simulink model "sschdlexFlybackConverterExample"  (R2023b)
settings: Solver=FixedStepDiscrete  StartTime=0.0  StopTime=200e-6  RelTol=1e-3
InitFcn:
  | ts = 2e-008;
libraries: fl_lib x13, nesl_utility x7, ee_lib x2, simulink x1, hdlsllib x1
CloseFcn:
  | clear ts;
settings Model: DataTypeOverride=Off  Creator=The MathWorks, Inc.  LastModifiedBy=The MathWorks, Inc.
settings SolverCC: AlgebraicLoopSolver=TrustRegion
settings OptimizationCC: BlockReduction=off  ConditionallyExecuteInputs=off  DefaultParameterBehavior=Inlined
settings DebuggingCC: AlgebraicLoopMsg=error  SingleTaskRateTransMsg=error  ParameterPrecisionLossMsg=none  UnconnectedInputMsg=warning  UnconnectedOutputMsg=warning  UnconnectedLineMsg=warning
settings HardwareCC: ProdBitPerPointer=32  ProdBitPerSizeT=32  ProdBitPerPtrDiffT=32  ProdLargestAtomicFloat=None  ProdIntDivRoundTo=Undefined  ProdEndianess=Unspecified  ProdWordSize=32  ProdHWDeviceType=ASIC/FPGA->ASIC/FPGA  TargetBitPerPointer=64  TargetBitPerSizeT=64  TargetBitPerPtrDiffT=64  TargetLongLongMode=on  TargetIntDivRoundTo=Zero  TargetEndianess=LittleEndian  TargetWordSize=64  TargetHWDeviceType=Custom Processor->MATLAB Host Computer  ProdEqTarget=off
settings ModelReferenceCC: EnableRefExpFcnMdlSchedulingChecks=on
settings RTWCC: DLArmComputeVersion=19.05

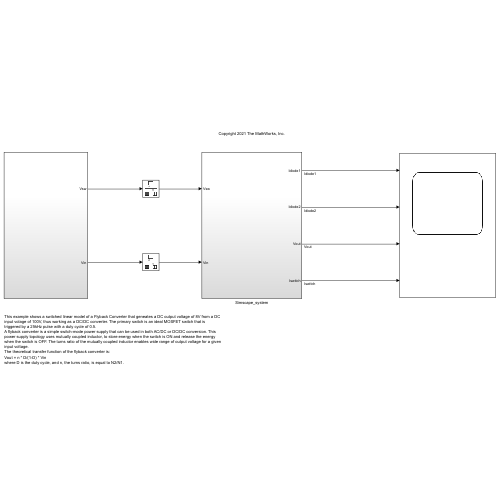
[thumbnail: Simulink's stored preview of the top-level diagram]
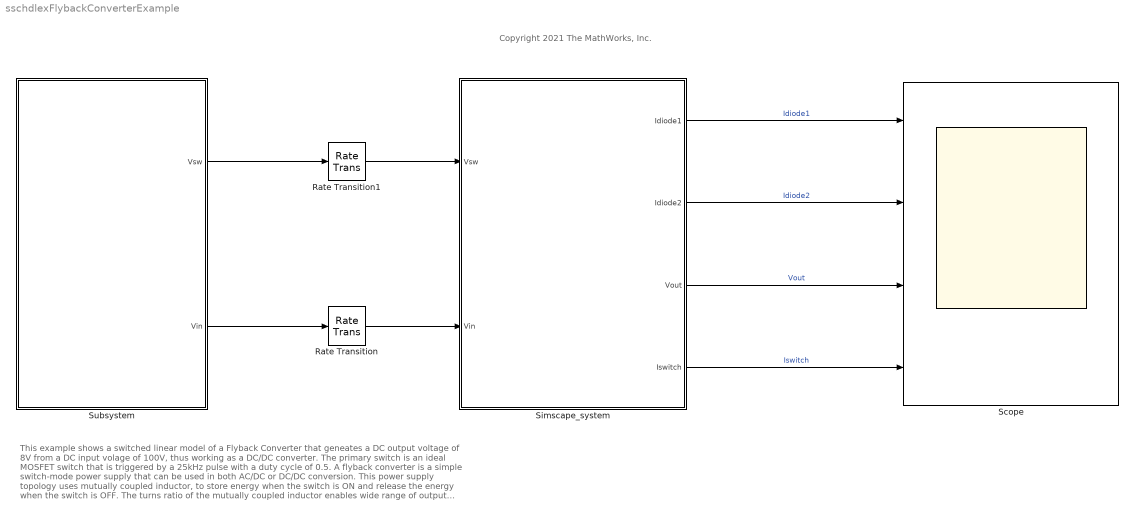
== system sschdlexFlybackConverterExample ==
  note: This example shows a switched linear model of a Flyback Converter that geneates a DC output voltage of 8V from a DC input volage of 100V, thus working as a DC/DC converter. The primary switch is an ideal MOSFET switch that is triggered by a 25kHz pulse with a duty cycle of 0.5.
      | A flyback converter is a simple switch-mode power supply that can be used in both AC/DC or DC/DC conversion. This power supply topology uses mutually coupled inductor, to store energy when the switch is ON and release the energy when the switch is OFF. The turns ratio of the mutually coupled inductor enables wide range of output voltage for a given input voltage.
      | The theoretical transfer function of the flyback converter is:
      | Vout = n * D/(1-D) * Vin
      | where D is the duty cycle, and n, the turns ratio, is equal to N2/N1.
  note: Copyright 2021 The MathWorks, Inc.
  Rate Transition : RateTransition
  Rate Transition1 : RateTransition
  Scope : Scope  NumInputPorts=4
  Simscape_system : Subsystem
  Subsystem : Subsystem
  wires:
  Subsystem/1(Vsw) -> Rate Transition1/1
  Subsystem/2(Vin) -> Rate Transition/1
  Rate Transition1/1 -> Simscape_system/1(Vsw)
  Rate Transition/1 -> Simscape_system/2(Vin)
  Simscape_system/1(Idiode1) -> Scope/1  "Idiode1"
  Simscape_system/2(Idiode2) -> Scope/2  "Idiode2"
  Simscape_system/3(Vout) -> Scope/3  "Vout"
  Simscape_system/4(Iswitch) -> Scope/4  "Iswitch"

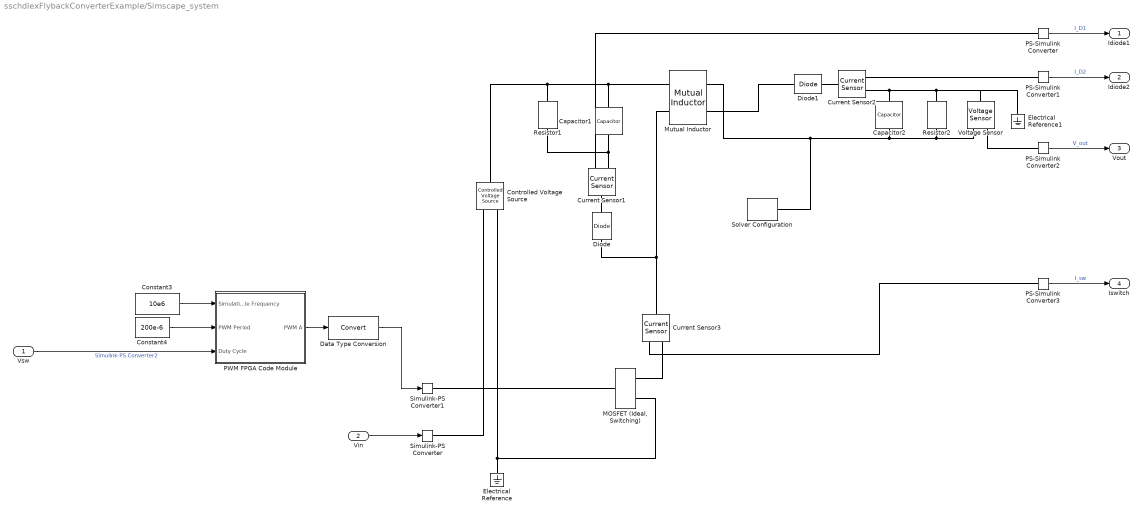
== system sschdlexFlybackConverterExample/Simscape_system ==
  Vsw : Inport
  Vin : Inport  Port=2
  Capacitor1 : fl_lib/Electrical/Electrical Elements/Capacitor  c=0.1e-12 F  r=0 Ohm  g=0 1/Ohm  i_specify=off  i_priority=None  i=0 A  i_nominal_specify=off  i_nominal_unit=A  i_nominal_value=1  v_specify=off  v_priority=None  v=0 V  v_nominal_specify=off  v_nominal_unit=V  v_nominal_value=1  vc_specify=off  vc_priority=High  vc=0 V  vc_nominal_specify=off  vc_nominal_unit=V  vc_nominal_value=1
  Capacitor2 : fl_lib/Electrical/Electrical Elements/Capacitor  c=50e-6 F  r=0 Ohm  g=0 1/Ohm  i_specify=off  i_priority=None  i=0 A  i_nominal_specify=off  i_nominal_unit=A  i_nominal_value=1  v_specify=off  v_priority=None  v=0 V  v_nominal_specify=off  v_nominal_unit=V  v_nominal_value=1  vc_specify=on  vc_priority=High  vc=8 V  vc_nominal_specify=off  vc_nominal_unit=V  vc_nominal_value=1
  Constant3 : Constant  Value=10e6  OutDataTypeStr=single  SampleTime=-1
  Constant4 : Constant  Value=200e-6  OutDataTypeStr=single  SampleTime=-1
  Controlled Voltage Source : fl_lib/Electrical/Electrical Sources/Controlled Voltage Source
  Current Sensor1 : fl_lib/Electrical/Electrical Sensors/Current Sensor
  Current Sensor2 : fl_lib/Electrical/Electrical Sensors/Current Sensor
  Current Sensor3 : fl_lib/Electrical/Electrical Sensors/Current Sensor
  Data Type Conversion : DataTypeConversion  SaturateOnIntegerOverflow=off  RndMeth=Floor
  Diode : fl_lib/Electrical/Electrical Elements/Diode  Vf=0.001 V  Ron=0.001 Ohm  Goff=1e-6 1/Ohm  i_specify=off  i_priority=None  i=0 A  i_nominal_specify=off  i_nominal_unit=A  i_nominal_value=1  v_specify=off  v_priority=None  v=0 V  v_nominal_specify=off  v_nominal_unit=V  v_nominal_value=1
  Diode1 : fl_lib/Electrical/Electrical Elements/Diode  Vf=0.25 V  Ron=0.3 Ohm  Goff=1e-8 1/Ohm  i_specify=off  i_priority=None  i=0 A  i_nominal_specify=off  i_nominal_unit=A  i_nominal_value=1  v_specify=off  v_priority=None  v=0 V  v_nominal_specify=off  v_nominal_unit=V  v_nominal_value=1
  Electrical Reference : fl_lib/Electrical/Electrical Elements/Electrical Reference
  Electrical Reference1 : fl_lib/Electrical/Electrical Elements/Electrical Reference
  "MOSFET (Ideal, Switching)" : ee_lib/Semiconductors & Converters/MOSFET (Ideal, Switching)  Rds=1e-9 Ohm  Goff=1e-9 1/Ohm  Vth=0.001 V  diode_param=1  diode_Vf=0.8 V  diode_Ron=0.001 Ohm  diode_Goff=1e-5 1/Ohm  diode_C=50e-9 F  diode_iRM=-235 A  diode_iF=300 A  diode_idot=-50 A/us  diode_trr_param=1  diode_trr_factor=3  diode_trr=15 us  diode_Qrr=1500 s*uA  thermal_loss_option=ee.enum.converters.thermalLossOption.constantvalues  Von_data=[0, 1.1, 1.3, 1.45, 1.75, 2.25, 2.7; 0, 1, 1.15, 1.35, 1.7, 2.35, 3] V  Eon_data=[0, .29, 1.43, 2.86, 5.71, 13.14, 22.86; 0, .57, 2.63, 5.14, 10.29, 20.57, 30.29] * 1e-3 J  Eoff_data=[0, .21, 1.07, 2.14, 4.29, 9.86, 17.14; 0, .43, 1.97, 3.86, 7.71, 15.43, 22.71] * 1e-3 J  Tj=[298.15, 398.15] K  Iout_data=[0, 10, 50, 100, 200, 400, 600] A  Eon_scalar=22.86e-3 J  Eoff_scalar=17.14e-3 J  Voff=300 V  Iout_scalar=600 A  diodeModelType=ee.enum.converters.diodeModelType.pwl  diode_IfMat=[.07, .12, .19, 1.75, 4.24, 7.32, 11.2; .16, .3, .72, 2.14, 4.02, 6.35, 9.12] A  diode_TjVec=[25, 125] degC  diode_VfVec=[.5, .7, .9, 1.3, 1.7, 2.1, 2.5] V  thermal_network_parameterization=ee.enum.thermalNetworkTopology.external  Rth=[.03, .2] K/W  Rth_Foster=[.03, .2] K/W  thermal_mass_parameterization=ee.enum.thermalNetwork.timeconstant  thermal_mass=[3, 25] J/K  thermal_mass_Foster=[33, 50] J/K  thermal_time_constant=[.1, 5] s  thermal_time_constant_Foster=[1, 10] s  thermal_mass_initial_temperatures=[25, 25] degC  junction_thermal_mass=0.1 J/K  Tau=1e-4 s  vT_specify=off  vT_priority=None  vT=0 V  vT_nominal_specify=off  vT_nominal_unit=V  vT_nominal_value=1  Qj_specify=off  Qj_priority=None  Qj=0 W  Qj_nominal_specify=off  Qj_nominal_unit=W  Qj_nominal_value=1  junction_temperature_specify=off  junction_temperature_priority=None  junction_temperature=25 degC  junction_temperature_nominal_specify=off  junction_temperature_nominal_unit=degC  junction_temperature_nominal_value=1
  Mutual Inductor : ee_lib/Passive/Transformers/Mutual Inductor  L1=10 uH  L2=10 uH  k=0.08  L_tol=5  enable_L1_tol=0  L1_tol_distribution=1  L1_nSigma=4  enable_L2_tol=0  L2_tol_distribution=1  L2_nSigma=4  r=[.1e-3, .1e-3] Ohm  g=[1e-09, 1e-09] 1/Ohm  enable_operating_limits=0  operating_limit_action=2  max_working_current=1 A  power_rating=1 W  enable_faults=ee.enum.faults.faultEnable.no  fault_action=ee.enum.faults.faultAction.none  fault_winding=1  lambdaPercent=50  turnsShort=ee.enum.faults.faultTurnsShort.no  openCct=ee.enum.faults.faultTurnsOpenCkt.no  groundShort=ee.enum.faults.faultTurnsGroundShort.no  groundShortG=0 1/Ohm  tau_fault=1e-3 s  enable_temporal_fault=ee.enum.faults.faultTriggerTemporal.no  t_fault=1 s  enable_behavioral_fault=ee.enum.faults.faultTriggerBehavioral.no  max_permissible_voltage=100 V  n_fail_on_voltage=1  max_permissible_current=1 A  t_fail_on_current=1 s  iL1_specify=off  iL1_priority=High  iL1=0 A  iL1_nominal_specify=off  iL1_nominal_unit=A  iL1_nominal_value=1  iL2_specify=off  iL2_priority=High  iL2=0 A  iL2_nominal_specify=off  iL2_nominal_unit=A  iL2_nominal_value=1
      settings: InternalSimscapePortConfiguration="{\"Bottom\":[],\"Left\":[{\"id\":\"p1\",\"label\":\"1+\",\"type\":\"foundation.electrical.electrical\"},{\"id\":\"n1\",\"label\":\"1-\",\"type\":\"foundation.electrical.electrical\"}],\"Right\":[{\"id\":\"p2\",\"label\":\"2+\",\"type\":\"foundation.electrical.electrical\"},{\"id\":\"n2\",\"label\":\"2-\",\"type\":\"foundation.electrical.electrical\"}],\"Top\":[]}"
  PS-Simulink Converter{,1..3} (4 alike) : nesl_utility/PS-Simulink Converter  PhysicalDomain=network_engine_domain  SubClassName=ps_output  LeftPortType=input  RightPortType=output  PseudoPeriodic=off  Frequencies=[]  Unit=inherit  AffineConversion=off
  PWM FPGA Code Module : Subsystem  SystemSampleTime=1/75e6
  Resistor1 : fl_lib/Electrical/Electrical Elements/Resistor  R=50e3 Ohm  i_specify=off  i_priority=None  i=0 A  i_nominal_specify=off  i_nominal_unit=A  i_nominal_value=1  v_specify=off  v_priority=None  v=0 V  v_nominal_specify=off  v_nominal_unit=V  v_nominal_value=1
  Resistor2 : fl_lib/Electrical/Electrical Elements/Resistor  R=2.5 Ohm  i_specify=off  i_priority=None  i=0 A  i_nominal_specify=off  i_nominal_unit=A  i_nominal_value=1  v_specify=off  v_priority=None  v=0 V  v_nominal_specify=off  v_nominal_unit=V  v_nominal_value=1
  Simulink-PS Converter : nesl_utility/Simulink-PS Converter  PhysicalDomain=network_engine_domain  SubClassName=ps_input  LeftPortType=input  RightPortType=output  PseudoPeriodic=off  Frequencies=[]  NoiseDistribution=none  NoiseParameters=[]  Unit=1  AffineConversion=off  FilteringAndDerivatives=provide  SimscapeFilterOrder=1  InputFilterTimeConstant=0.001  UdotUserProvided=0
  Simulink-PS Converter1 : nesl_utility/Simulink-PS Converter  PhysicalDomain=network_engine_domain  SubClassName=ps_input  LeftPortType=input  RightPortType=output  PseudoPeriodic=off  Frequencies=[]  NoiseDistribution=none  NoiseParameters=[]  Unit=1  AffineConversion=off  FilteringAndDerivatives=provide  SimscapeFilterOrder=1  InputFilterTimeConstant=0.001  UdotUserProvided=0
  Solver Configuration : nesl_utility/Solver Configuration  PhysicalDomain=network_engine_domain  SubClassName=solver  LeftPortType=input  RightPortType=generic  Tones=[]  Harmonics=[]  SimulateNoise=off  Profile=off  UseLocalSampling=off  EnableSwitchedLinearOptims=on  FrequencyDomain=off  UseCCode=off  RelTol=0.001  AbsTol=1e-06  MinStep=1e-09  ToWorkspace=off  RevertToSquareIcSolve=off  NumHomotopyIterations=100  PhasorMode=off  PhasorModeNumHarmonics=1  DoDC=off  ResidualTolerance=1e-09  UseLocalSolver=on  LocalSolverChoice=NE_BACKWARD_EULER_ADVANCER  LocalSolverSampleTime=ts  DoFixedCost=on  MaxNonlinIter=3  MaxModeIter=2  ComputeImpulses=off  ImpulseIterations=1  LinearAlgebra=auto  EquationFormulation=NE_TIME_EF  DelaysMemoryBudget=1024  AutomaticFiltering=on  FilteringTimeConstant=0.001  PartitionStorageMethod=AS_NEEDED  PartitionMemoryBudget=1024  PartitionMethod=ROBUST
  Voltage Sensor : fl_lib/Electrical/Electrical Sensors/Voltage Sensor
  Idiode1 : Outport
  Idiode2 : Outport  Port=2
  Vout : Outport  Port=3
  Iswitch : Outport  Port=4
  wires:
  Data Type Conversion/1 -> Simulink-PS Converter1/1
  Vin/1 -> Simulink-PS Converter/1
  PS-Simulink Converter2/1 -> Vout/1  "V_out"
  PS-Simulink Converter1/1 -> Idiode2/1  "I_D2"
  PS-Simulink Converter/1 -> Idiode1/1  "I_D1"
  PS-Simulink Converter3/1 -> Iswitch/1  "I_sw"
  Vsw/1 -> PWM FPGA Code Module/3(Duty Cycle)  "Simulink-PS Converter2"
  Constant4/1 -> PWM FPGA Code Module/2(PWM Period)
  PWM FPGA Code Module/1(PWM A) -> Data Type Conversion/1
  Constant3/1 -> PWM FPGA Code Module/1(Simulation Sample Frequency)
  connections:
  Diode/RConn1 -- Current Sensor1/LConn1
  Electrical Reference/LConn1 -- "MOSFET (Ideal, Switching)"/RConn2 -- Controlled Voltage Source/RConn2
  "MOSFET (Ideal, Switching)"/LConn1 -- Simulink-PS Converter1/RConn1
  Capacitor1/RConn1 -- Resistor1/RConn1 -- Current Sensor1/RConn2
  Current Sensor3/LConn1 -- Diode/LConn1 -- Mutual Inductor/LConn2
  Current Sensor1/RConn1 -- PS-Simulink Converter/LConn1
  Diode1/RConn1 -- Current Sensor2/LConn1
  PS-Simulink Converter2/LConn1 -- Voltage Sensor/RConn1
  Current Sensor2/RConn2 -- Capacitor2/LConn1 -- Resistor2/LConn1 -- Electrical Reference1/LConn1 -- Voltage Sensor/LConn1
  Simulink-PS Converter/RConn1 -- Controlled Voltage Source/RConn1
  Controlled Voltage Source/LConn1 -- Resistor1/LConn1 -- Mutual Inductor/LConn1 -- Capacitor1/LConn1
  Solver Configuration/RConn1 -- Mutual Inductor/RConn1 -- Capacitor2/RConn1 -- Resistor2/RConn1 -- Voltage Sensor/RConn2
  PS-Simulink Converter1/LConn1 -- Current Sensor2/RConn1
  PS-Simulink Converter3/LConn1 -- Current Sensor3/RConn1
  Current Sensor3/RConn2 -- "MOSFET (Ideal, Switching)"/RConn1
  Diode1/LConn1 -- Mutual Inductor/RConn2

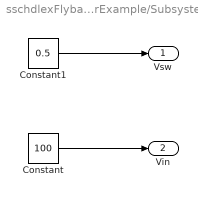
== system sschdlexFlybackConverterExample/Subsystem ==
  Constant : Constant  Value=100  SampleTime=0
  Constant1 : Constant  Value=0.5  SampleTime=ts
  Vsw : Outport
  Vin : Outport  Port=2
  wires:
  Constant1/1 -> Vsw/1
  Constant/1 -> Vin/1

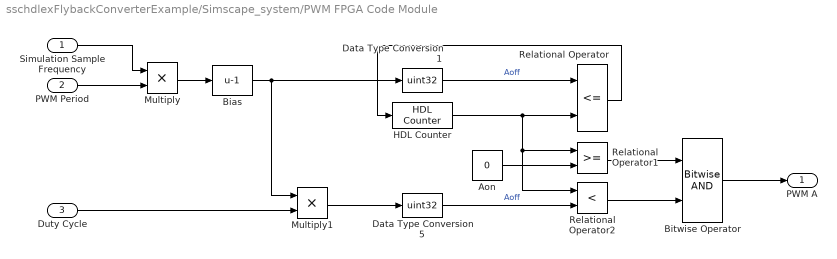
== system sschdlexFlybackConverterExample/Simscape_system/PWM FPGA Code Module ==
  Simulation Sample Frequency : Inport
  PWM Period : Inport  Port=2
  Duty Cycle : Inport  Port=3
  Aon : Constant  Value=0  OutDataTypeStr=uint32  SampleTime=-1
  Bias : Bias  Bias=-1  SaturateOnIntegerOverflow=off
  Bitwise Operator : simulink/Logic and Bit Operations/Bitwise Operator  logicop=AND  UseBitMask=off  NumInputPorts=2  BitMask=bin2dec('11011001')  BitMaskRealWorld=Stored Integer
  Data Type Conversion1 : DataTypeConversion  OutDataTypeStr=uint32  SaturateOnIntegerOverflow=off  RndMeth=Floor
  Data Type Conversion5 : DataTypeConversion  OutDataTypeStr=uint32  SaturateOnIntegerOverflow=off  RndMeth=Floor
  HDL Counter : hdlsllib/Sources/HDL Counter  CountType=Free running  CountInit=0  CountStep=1  CountMax=25  CountFromType=Initial value  CountFrom=0  CountResetPort=on  CountLoadPort=off  CountEnbPort=off  CountDirPort=off  CountHitOutputPort=off  CountDataType=Unsigned  CountWordLen=32  CountFracLen=0  CountSampTime=1
  Multiply : Product
  Multiply1 : Product
  Relational Operator : RelationalOperator  Operator=<=  OutDataTypeStr=boolean  InputSameDT=off
  Relational Operator1 : RelationalOperator  OutDataTypeStr=boolean  InputSameDT=off
  Relational Operator2 : RelationalOperator  Operator=<  OutDataTypeStr=boolean  InputSameDT=off
  PWM A : Outport  VectorParamsAs1DForOutWhenUnconnected=off
  wires:
  Bias/1 -> Data Type Conversion1/1, Multiply1/1
  Relational Operator/1 -> HDL Counter/1
  Aon/1 -> Relational Operator1/2
  Data Type Conversion5/1 -> Relational Operator2/2  "Aoff"
  Relational Operator1/1 -> Bitwise Operator/1
  Relational Operator2/1 -> Bitwise Operator/2
  Bitwise Operator/1 -> PWM A/1
  HDL Counter/1 -> Relational Operator2/1, Relational Operator1/1, Relational Operator/2
  PWM Period/1 -> Multiply/2
  Multiply/1 -> Bias/1
  Multiply1/1 -> Data Type Conversion5/1
  Simulation Sample Frequency/1 -> Multiply/1
  Duty Cycle/1 -> Multiply1/2
  Data Type Conversion1/1 -> Relational Operator/1  "Aoff"
